simulink library "SimFly_Serial"  (R2015b)
settings: Solver=VariableStepAuto  StartTime=0.0  StopTime=10.0  RelTol=1e-3
settings Model: Creator=mocherma  LastModifiedBy=marcell

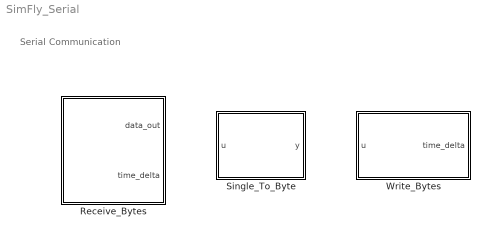
== system SimFly_Serial ==
  note: Serial Communication
  Receive_Bytes : MATLAB Function  TreatAsAtomicUnit=on
  Single_To_Byte : MATLAB Function  TreatAsAtomicUnit=on
  Write_Bytes : MATLAB Function  TreatAsAtomicUnit=on

== matlab function SimFly_Serial/Receive_Bytes ==
  settings: updateMethod=DISCRETE  sampleTime=1/1000
  data: data_out output; time_delta output
function [data_out,time_delta]  = data_receive()
%PURPOSE: (Example) Driver for serial_receive from instrument toolbox
%AUTHOR: Marcell Mocher
%DATE: 3.1.2017
%VERSION: 0.1 V Fist build
%Input: -
%Output: data_out = 
%Info: This drive requires function call triggered simuluink functions in
% order to work
%Requires:  _get_time
%           _serial_init
%           _serial_available
%           _serial_read

persistent init_flag alive_flag state head_count idx data length


data_out = single(zeros(64,1));

if strcmp(coder.target, 'rtw'),
  
time_start = uint32(0);
time_start = coder.ceval('_get_time');

% Parameter from Mask!
baud = uint32(115200); 


% Init parameters

if isempty(init_flag)
    init_flag = 0;
    alive_flag = true;
    length = uint8(1);
    data = uint8(zeros(512,1));
    idx = uint8(1);
    state = uint8(0);
    head_count = uint8(0);
    coder.ceval('_serial_init',uint8(0),baud);   
    coder.ceval('_serial_init',uint8(1),baud);  
end

av = uint8(0);
av = coder.ceval('_serial_available',uint8(0));
if av > 0
    for i = 1:av
        cc = uint8(0);
        cc = coder.ceval('_serial_read',uint8(0));
        switch state
            case 0 %wait for sync 1 (98)
                if cc == 98 
                    state = state + 1;
                    head_count = uint8(1);
                end
            case 1 %wait for sync 1 (98)
                if cc == 98
                    head_count = head_count + 1;
                    if head_count >= 4
                        state = state + 1;
                        idx = uint8(1);
                    end
                else
                    state = uint8(0);
                    head_count = uint8(0);
                end
            case 2 %wait for length
                length = cc;
                state = state + 1;
            case 3 %wait for values
                data(idx) = cc;
                idx = idx + 1;
                if idx > length
                    state = uint8(0);
                end
        end % End of switch (state)
        
    end % End for
    
end % End if

data_out(1:length/4) = typecast(data(1:length),'single');

time_end = uint32(0);
time_end = coder.ceval('_get_time');
time_delta = time_end - time_start;

%coder.ceval('_serial_print',uint8(1),double(data_out(4)));
%coder.ceval('_serial_print',uint8(1),double(0));
else
alive = true;  %TODO: alive flag impementation
time_delta = uint32(0);
end
end

== matlab function SimFly_Serial/Write_Bytes ==
  data: u input; time_delta output
function time_delta = write(u)
%PURPOSE: (Example) Driver for Serial writing with hardware abstraction layer
%AUTHOR: Marcell Mocher
%DATE: 3.1.2017
%VERSION: 0.1 V Fist build
%Input: Array to print on the serial port
%Output: Execution time
%Info: This drive requires function call triggered simuluink functions in
% order to work
%Requires:  _get_time
%           _serial_init
%           _serial_print
%           _serial_write
persistent init_flag

if strcmp(coder.target, 'rtw'),
    
    time_start = uint32(0);
    time_start = coder.ceval('_get_time');
    
    if isempty(init_flag)
        init_flag = true;
        coder.ceval('_serial_init',uint8(0),uint32(115200));
    end
    len = uint8(numel(u));
    coder.ceval('_serial_write',uint8(0),u,len);
    
    time_end = uint32(0);
    time_end = coder.ceval('_get_time');
    time_delta = time_end - time_start;
else
    time_delta = uint32(0);
end

== matlab function SimFly_Serial/Single_To_Byte ==
  data: u input; y output
function y = SingleToByte(u)
%PURPOSE: (Example) Convertion of single values to a binary array with header and
%terminator
%AUTHOR: Marcell Mocher
%DATE: 3.1.2017
%VERSION: 0.1 V Fist build
%Input: Array of single datatype values
%Output: 

% make sure we're calculating with single 
u = single(u);
% define header %
header = uint8(ones(8,1)*97);
% define terminator %
terminator = uint8([13;10]);

len = numel(u);
% we only have singles%
len_byte = len * 4;
y = uint8(zeros(len_byte+numel(header)+numel(terminator),1));
u_byte = typecast(u,'uint8');
y(1:numel(header)) = header;
for i = 1:numel(u_byte)
   y(i+numel(header)) = u_byte(i) ;
end
y(end-numel(terminator)+1:end) = terminator;
